simulink model "PubIfDecisionLM_MDL"  (R2020b)
settings: configuration reference "DspaceConfig" (kept outside this file)
PostLoadFcn:
  | if any(exist('dsrtsu_mdlpostloadfcn', 'file') ~= 0), dsrtsu_mdlpostloadfcn('Execute', bdroot); end
InitFcn:
  | , if any(exist('dsmpb_private', 'file') ~= 0), dsmpb_private('dsmpb_mdlclblib', 'Init', bdroot); end,
undefined symbols (not defined in the file or in its folder): OFM_OBJ_FUSIONTYPE_E, OFM_OBJ_MOVINGSTATE_E, OFM_OBJ_ORIENTATION_E, OFM_OBJ_TYPE_E, P_LM_Cyc, P_LM_EMLHistKapRcdBufSize, P_LM_EMLHistTrajBaseDis, P_LM_EMLHistTrajPNum, P_LM_EMLKapCorrMaxThre, P_LM_EMLMinKapThre, P_LM_EMLPathDisDiffThre, P_LM_EMLQuaFiltPar, P_LM_EMLTurnActKapThre, P_LM_EMLValidQuaThre, P_LM_FntPath1Disgap, P_LM_FntPath1MinDis, P_LM_FntPath1Timegap, P_LM_FntPath2Disgap, P_LM_FntPath2MinDis, P_LM_FntPath2Timegap, P_LM_FntPath3Disgap, P_LM_FntPath3MinDis, P_LM_FntPath3Timegap, P_LM_FusBLParFiltP, P_LM_FusEVDifC2Thre, P_LM_FusEVOPath1AllVSLDisThre, P_LM_FusEVOPath1AllVSLLostNumThre, P_LM_FusEVOPath1AllVSLQuaThre, P_LM_FusEVOPath1OTLFacNLC, P_LM_FusOTLQuaThre, P_LM_FusOTLSW, P_LM_FusParC0Index, P_LM_FusParC1Index, P_LM_FusParC2Index, P_LM_FusParC3Index, P_LM_FusVSLQuaThre, P_LM_FusVSLSW, P_LM_FusVSLValidSteerWheerAngThre, P_LM_FusVSLValidVxvThre, P_LM_LaneWidth, P_LM_OTLBufTPInfoEvaFactor, P_LM_OTLObjNum, P_LM_OTLObjSelectAgeThre, P_LM_OTLObjSelectDxAssessVx, P_LM_OTLObjSelectDxThre, P_LM_OTLObjSelectVxThre, P_LM_OTLObjSelectVyAssessDx, P_LM_OTLObjSelectVyThre, P_LM_OTLTrajPntBaseDis, P_LM_OTLTrajStdThre, P_LM_VSLAvailLineNum, P_LM_VSLBLSDiffThre, P_LM_VSLBLSDisRatio, P_LM_VSLFusBLParFiltP_C1, P_LM_VSLFusBLParFiltP_C2, P_LM_VSLFusBLParFiltP_C3, P_LM_VSLFusBLParFiltP_Quality, P_LM_VSLHistTrajBaseDis, P_LM_VSLHistTrajPNum, P_LM_VSLLCC0diff ... (+18)
libraries: simulink x145, LM_LIB x43
(part 19 of 24)

== system PubIfDecisionLM_MDL/Subsystem2/LM_Fusion1/LM_FusRatioCalc/LM_Fusion_EVO/LM_FusEVORatioCalc/LM_Fusion_FntPathK/LM_FusEVOFntPath3/If Action Subsystem1/Subsystem ==
  LM_FusEVOFntPath3EMLFac : Inport
  LM_FusEVOFntPath3VSLFac : Inport  Port=2
  LM_FusEVOFntPath3OTLFac : Inport  Port=3
  LM_EMLFntPath3Quality : Inport  Port=4
  LM_VSLFntPath3Quality : Inport  Port=5
  LM_OTLFntPath3Qulity : Inport  Port=6
  Add : Sum
  Add1 : Sum
  Compare To Zero : simulink/Logic and Bit Operations/Compare To Zero  relop===  OutDataTypeStr=boolean
  Constant : Constant  Value=0.000001  OutDataTypeStr=single
  Divide : Product  Inputs=*/
  Divide1 : Product  Inputs=*/
  Divide2 : Product  Inputs=*/
  Product : Product
  Product1 : Product
  Product2 : Product
  Switch : Switch  Criteria=u2 ~= 0
  LM_FusEVOFntPath3EMLK : Outport
  LM_FusEVOFntPath3VSLK : Outport  Port=2
  LM_FusEVOFntPath3OTLK : Outport  Port=3
  wires:
  Divide1/1 -> LM_FusEVOFntPath3VSLK/1  "LM_FusEVOFntPath3VSLK"
  Divide2/1 -> LM_FusEVOFntPath3OTLK/1  "LM_FusEVOFntPath3OTLK"
  Product/1 -> Divide/1, Add/1
  Add/1 -> Add1/1
  Switch/1 -> Divide2/2, Divide1/2, Divide/2
  Product2/1 -> Divide2/1, Add1/2
  Divide/1 -> LM_FusEVOFntPath3EMLK/1  "LM_FusEVOFntPath3EMLK"
  Product1/1 -> Add/2, Divide1/1
  LM_FusEVOFntPath3OTLFac/1 -> Product2/2
  LM_FusEVOFntPath3VSLFac/1 -> Product1/2
  LM_FusEVOFntPath3EMLFac/1 -> Product/2
  LM_OTLFntPath3Qulity/1 -> Product2/1
  LM_VSLFntPath3Quality/1 -> Product1/1
  LM_EMLFntPath3Quality/1 -> Product/1
  Add1/1 -> Switch/3, Compare To Zero/1
  Compare To Zero/1 -> Switch/2
  Constant/1 -> Switch/1

== system PubIfDecisionLM_MDL/Subsystem2/LM_OTL/LM_OTL_MovObjTrajRecord3/LM_OTL_BufTPCC/Subsystem/LM_OTLHostBufCoordinateConvert/If Action Subsystem/For Each Subsystem/LM_VSL_BufE1Convert ==
  LM_OTLBufE1DxVectK1 : Inport
  LM_OTLBufE1DyVectK1 : Inport  Port=2
  LM_EgoVehOffsetX : Inport  Port=3
  LM_EgoVehOffsetY : Inport  Port=4
  LM_EgoVehOffsetAng : Inport  Port=5
  Add : Sum
  Product{,1..3} (4 alike) : Product
  Sin : Trigonometry
  Sin1 : Trigonometry  Operator=cos
  Subtract : Sum  Inputs=+-
  Subtract1 : Sum  Inputs=+-
  Subtract2 : Sum  Inputs=+-
  LM_OTLBufE1DxVectK1Adju : Outport
  LM_OTLBufE1DyVectK1Adju : Outport  Port=2
  wires:
  Subtract1/1 -> Product3/1, Product1/1
  Sin1/1 -> Product3/2, Product/2
  Product2/1 -> Add/1
  Product/1 -> Subtract2/1
  Product1/1 -> Subtract2/2
  LM_OTLBufE1DyVectK1/1 -> Subtract1/1
  LM_EgoVehOffsetAng/1 -> Sin1/1, Sin/1
  Sin/1 -> Product2/2, Product1/2
  Subtract/1 -> Product2/1, Product/1
  Product3/1 -> Add/2
  Add/1 -> LM_OTLBufE1DyVectK1Adju/1  "LM_OTLBufE1DyVectK1Adju"
  LM_OTLBufE1DxVectK1/1 -> Subtract/1
  LM_EgoVehOffsetY/1 -> Subtract1/2
  LM_EgoVehOffsetX/1 -> Subtract/2
  Subtract2/1 -> LM_OTLBufE1DxVectK1Adju/1  "LM_OTLBufE1DxVectK1Adju"

== system PubIfDecisionLM_MDL/Subsystem2/LM_OTL/LM_OTL_MovObjTrajRecord3/LM_OTL_BufTPCC/Subsystem/LM_OTLHostBufCoordinateConvert/If Action Subsystem/For Each Subsystem/LM_VSL_BufE2Convert ==
  LM_OTLBufE2DxVectK1 : Inport
  LM_OTLBufE2DyVectK1 : Inport  Port=2
  LM_EgoVehOffsetX : Inport  Port=3
  LM_EgoVehOffsetY : Inport  Port=4
  LM_EgoVehOffsetAng : Inport  Port=5
  Add : Sum
  Product{,1..3} (4 alike) : Product
  Sin : Trigonometry
  Sin1 : Trigonometry  Operator=cos
  Subtract : Sum  Inputs=+-
  Subtract1 : Sum  Inputs=+-
  Subtract2 : Sum  Inputs=+-
  LM_OTLBufE2DxVectK1Adju : Outport
  LM_OTLBufE2DyVectK1Adju : Outport  Port=2
  wires:
  Subtract2/1 -> LM_OTLBufE2DxVectK1Adju/1  "LM_OTLBufE2DxVectK1Adju"
  LM_EgoVehOffsetX/1 -> Subtract/2
  LM_EgoVehOffsetY/1 -> Subtract1/2
  LM_OTLBufE2DxVectK1/1 -> Subtract/1
  Add/1 -> LM_OTLBufE2DyVectK1Adju/1  "LM_OTLBufE2DyVectK1Adju"
  Product3/1 -> Add/2
  Subtract/1 -> Product/1, Product2/1
  Sin/1 -> Product1/2, Product2/2
  LM_EgoVehOffsetAng/1 -> Sin/1, Sin1/1
  LM_OTLBufE2DyVectK1/1 -> Subtract1/1
  Product1/1 -> Subtract2/2
  Product/1 -> Subtract2/1
  Product2/1 -> Add/1
  Sin1/1 -> Product/2, Product3/2
  Subtract1/1 -> Product1/1, Product3/1

== system PubIfDecisionLM_MDL/Subsystem2/LM_OTL/LM_OTL_MovObjTrajRecord3/LM_OTL_BufTPCC/Subsystem/LM_OTLLeBufCoordinateConvert/If Action Subsystem/For Each Subsystem/LM_OTL_BufL1Convert ==
  LM_OTLBufL1DxVectK1 : Inport
  LM_OTLBufL1DyVectK1 : Inport  Port=2
  LM_EgoVehOffsetX : Inport  Port=3
  LM_EgoVehOffsetY : Inport  Port=4
  LM_EgoVehOffsetAng : Inport  Port=5
  Add : Sum
  Product{,1..3} (4 alike) : Product
  Sin : Trigonometry
  Sin1 : Trigonometry  Operator=cos
  Subtract : Sum  Inputs=+-
  Subtract1 : Sum  Inputs=+-
  Subtract2 : Sum  Inputs=+-
  LM_OTLBufL1DxVectK1Adju : Outport
  LM_OTLBufL1DyVectK1Adju : Outport  Port=2
  wires:
  Subtract1/1 -> Product3/1, Product1/1
  Sin1/1 -> Product3/2, Product/2
  Product2/1 -> Add/1
  Product/1 -> Subtract2/1
  Product1/1 -> Subtract2/2
  LM_OTLBufL1DyVectK1/1 -> Subtract1/1
  LM_EgoVehOffsetAng/1 -> Sin1/1, Sin/1
  Sin/1 -> Product2/2, Product1/2
  Subtract/1 -> Product2/1, Product/1
  Product3/1 -> Add/2
  Add/1 -> LM_OTLBufL1DyVectK1Adju/1  "LM_OTLBufL1DyVectK1Adju"
  LM_OTLBufL1DxVectK1/1 -> Subtract/1
  LM_EgoVehOffsetY/1 -> Subtract1/2
  LM_EgoVehOffsetX/1 -> Subtract/2
  Subtract2/1 -> LM_OTLBufL1DxVectK1Adju/1  "LM_OTLBufL1DxVectK1Adju"

== system PubIfDecisionLM_MDL/Subsystem2/LM_OTL/LM_OTL_MovObjTrajRecord3/LM_OTL_BufTPCC/Subsystem/LM_OTLLeBufCoordinateConvert/If Action Subsystem/For Each Subsystem/LM_VSL_BufL2Convert ==
  LM_OTLBufL2DxVectK1 : Inport
  LM_OTLBufL2DyVectK1 : Inport  Port=2
  LM_EgoVehOffsetX : Inport  Port=3
  LM_EgoVehOffsetY : Inport  Port=4
  LM_EgoVehOffsetAng : Inport  Port=5
  Add : Sum
  Product{,1..3} (4 alike) : Product
  Sin : Trigonometry
  Sin1 : Trigonometry  Operator=cos
  Subtract : Sum  Inputs=+-
  Subtract1 : Sum  Inputs=+-
  Subtract2 : Sum  Inputs=+-
  LM_OTLBufL2DxVectK1Adju : Outport
  LM_OTLBufL2DyVectK1Adju : Outport  Port=2
  wires:
  Subtract2/1 -> LM_OTLBufL2DxVectK1Adju/1  "LM_OTLBufL2DxVectK1Adju"
  LM_EgoVehOffsetX/1 -> Subtract/2
  LM_EgoVehOffsetY/1 -> Subtract1/2
  LM_OTLBufL2DxVectK1/1 -> Subtract/1
  Add/1 -> LM_OTLBufL2DyVectK1Adju/1  "LM_OTLBufL2DyVectK1Adju"
  Product3/1 -> Add/2
  Subtract/1 -> Product/1, Product2/1
  Sin/1 -> Product1/2, Product2/2
  LM_EgoVehOffsetAng/1 -> Sin/1, Sin1/1
  LM_OTLBufL2DyVectK1/1 -> Subtract1/1
  Product1/1 -> Subtract2/2
  Product/1 -> Subtract2/1
  Product2/1 -> Add/1
  Sin1/1 -> Product/2, Product3/2
  Subtract1/1 -> Product1/1, Product3/1

== system PubIfDecisionLM_MDL/Subsystem2/LM_OTL/LM_OTL_MovObjTrajRecord3/LM_OTL_BufTPCC/Subsystem/LM_OTLRiBufCoordinateConvert/If Action Subsystem/For Each Subsystem/LM_VSL_BufR1Convert ==
  LM_OTLBufR1DxVectK1 : Inport
  LM_OTLBufR1DyVectK1 : Inport  Port=2
  LM_EgoVehOffsetX : Inport  Port=3
  LM_EgoVehOffsetY : Inport  Port=4
  LM_EgoVehOffsetAng : Inport  Port=5
  Add : Sum
  Product{,1..3} (4 alike) : Product
  Sin : Trigonometry
  Sin1 : Trigonometry  Operator=cos
  Subtract : Sum  Inputs=+-
  Subtract1 : Sum  Inputs=+-
  Subtract2 : Sum  Inputs=+-
  LM_OTLBufR1DxVectK1Adju : Outport
  LM_OTLBufR1DyVectK1Adju : Outport  Port=2
  wires:
  Subtract1/1 -> Product3/1, Product1/1
  Sin1/1 -> Product3/2, Product/2
  Product2/1 -> Add/1
  Product/1 -> Subtract2/1
  Product1/1 -> Subtract2/2
  LM_OTLBufR1DyVectK1/1 -> Subtract1/1
  LM_EgoVehOffsetAng/1 -> Sin1/1, Sin/1
  Sin/1 -> Product2/2, Product1/2
  Subtract/1 -> Product2/1, Product/1
  Product3/1 -> Add/2
  Add/1 -> LM_OTLBufR1DyVectK1Adju/1  "LM_OTLBufR1DyVectK1Adju"
  LM_OTLBufR1DxVectK1/1 -> Subtract/1
  LM_EgoVehOffsetY/1 -> Subtract1/2
  LM_EgoVehOffsetX/1 -> Subtract/2
  Subtract2/1 -> LM_OTLBufR1DxVectK1Adju/1  "LM_OTLBufR1DxVectK1Adju"

== system PubIfDecisionLM_MDL/Subsystem2/LM_OTL/LM_OTL_MovObjTrajRecord3/LM_OTL_BufTPCC/Subsystem/LM_OTLRiBufCoordinateConvert/If Action Subsystem/For Each Subsystem/LM_VSL_BufR2Convert ==
  LM_OTLBufR2DxVectK1 : Inport
  LM_OTLBufR2DyVectK1 : Inport  Port=2
  LM_EgoVehOffsetX : Inport  Port=3
  LM_EgoVehOffsetY : Inport  Port=4
  LM_EgoVehOffsetAng : Inport  Port=5
  Add : Sum
  Product{,1..3} (4 alike) : Product
  Sin : Trigonometry
  Sin1 : Trigonometry  Operator=cos
  Subtract : Sum  Inputs=+-
  Subtract1 : Sum  Inputs=+-
  Subtract2 : Sum  Inputs=+-
  LM_OTLBufR2DxVectK1Adju : Outport
  LM_OTLBufR2DyVectK1Adju : Outport  Port=2
  wires:
  Subtract2/1 -> LM_OTLBufR2DxVectK1Adju/1  "LM_OTLBufR2DxVectK1Adju"
  LM_EgoVehOffsetX/1 -> Subtract/2
  LM_EgoVehOffsetY/1 -> Subtract1/2
  LM_OTLBufR2DxVectK1/1 -> Subtract/1
  Add/1 -> LM_OTLBufR2DyVectK1Adju/1  "LM_OTLBufR2DyVectK1Adju"
  Product3/1 -> Add/2
  Subtract/1 -> Product/1, Product2/1
  Sin/1 -> Product1/2, Product2/2
  LM_EgoVehOffsetAng/1 -> Sin/1, Sin1/1
  LM_OTLBufR2DyVectK1/1 -> Subtract1/1
  Product1/1 -> Subtract2/2
  Product/1 -> Subtract2/1
  Product2/1 -> Add/1
  Sin1/1 -> Product/2, Product3/2
  Subtract1/1 -> Product1/1, Product3/1

== system PubIfDecisionLM_MDL/Subsystem2/LM_OTL/LM_OTL_MovObjTrajRecord3/LM_OTL_MovObjSelc/LM_OTL_MovObjInterestedSelc/LM_OTL_ObjSelcIndexCalc/LM_OTL_ObjSelcCalc/LM_OTL_HostObjSelc/LM_OTL_HostObj1Selc ==
  C_LM_ObjNum : Inport
  In4 : Inport  Port=2
  Compare To Constant : simulink/Logic and Bit Operations/Compare To Constant  relop===  const=1  OutDataTypeStr=boolean
  Relational Operator : RelationalOperator  Operator=<  OutDataTypeStr=boolean  RndMeth=Simplest
  Switch : Switch  Criteria=u2 > Threshold
  Switch2 : Switch  Criteria=u2 ~= 0
  Switch28 : Switch  Criteria=u2 ~= 0
  Switch5 : Switch  Criteria=u2 > Threshold
  Unit Delay : UnitDelay  SampleTime=-1  HasFrameUpgradeWarning=on
  Unit Delay2 : UnitDelay  InitialCondition=255  SampleTime=-1  HasFrameUpgradeWarning=on
  LM_OTLHostObj1Index : Outport
  HostObj2SelcTrig : Outport  Port=2
  HostObj2SelcIndexPro : Outport  Port=3
  HostObj2SelcDxPro : Outport  Port=4
  wires:
  Compare To Constant/1 -> Switch28/2, Switch/2
  Relational Operator/1 -> Switch5/2, Switch2/2, HostObj2SelcTrig/1
  Switch28/1 -> Switch2/3
  In4/1 -> Relational Operator/1, Switch5/1, Switch/1
  C_LM_ObjNum/1 -> Compare To Constant/1, Switch2/1, Switch28/1
  Switch/1 -> Unit Delay2/1
  Switch2/1 -> Unit Delay/1, LM_OTLHostObj1Index/1
  Switch5/1 -> Switch/3
  Unit Delay/1 -> HostObj2SelcIndexPro/1, Switch28/3
  Unit Delay2/1 -> Switch5/3, HostObj2SelcDxPro/1, Relational Operator/2

== system PubIfDecisionLM_MDL/Subsystem2/LM_OTL/LM_OTL_MovObjTrajRecord3/LM_OTL_MovObjSelc/LM_OTL_MovObjInterestedSelc/LM_OTL_ObjSelcIndexCalc/LM_OTL_ObjSelcCalc/LM_OTL_HostObjSelc/LM_OTL_HostObj2Selc ==
  HostObj2SelcTrig : Inport
  HostObj2SelcIndexPro : Inport  Port=2
  HostObj2SelcDxPro : Inport  Port=3
  LM_OTL_HostObjSelcDxInfo : Inport  Port=4
  C_LM_ObjNum : Inport  Port=5
  Compare To Constant : simulink/Logic and Bit Operations/Compare To Constant  relop===  const=1  OutDataTypeStr=boolean
  Constant10 : Constant  Value=0  OutDataTypeStr=int32
  Constant8 : Constant  Value=255  OutDataTypeStr=single
  Relational Operator3 : RelationalOperator  Operator=<  OutDataTypeStr=boolean  RndMeth=Simplest
  Switch{20..22,26..27} (5 alike) : Switch  Criteria=u2 > Threshold
  Switch3 : Switch  Criteria=u2 ~= 0
  Unit Delay1 : UnitDelay  SampleTime=-1  HasFrameUpgradeWarning=on
  Unit Delay9 : UnitDelay  InitialCondition=255  SampleTime=-1  HasFrameUpgradeWarning=on
  LM_OTLLeObj2Index : Outport
  wires:
  HostObj2SelcDxPro/1 -> Switch20/1
  HostObj2SelcIndexPro/1 -> Switch3/1
  Constant10/1 -> Switch26/1
  Switch20/1 -> Switch21/3
  Switch27/1 -> Switch3/3
  Unit Delay1/1 -> Switch27/3
  Switch3/1 -> Switch26/3
  Unit Delay9/1 -> Switch22/3, Relational Operator3/2
  Constant8/1 -> Switch21/1
  HostObj2SelcTrig/1 -> Switch3/2, Switch20/2
  Relational Operator3/1 -> Switch22/2, Switch27/2
  C_LM_ObjNum/1 -> Switch27/1, Compare To Constant/1
  Switch26/1 -> LM_OTLLeObj2Index/1, Unit Delay1/1
  Compare To Constant/1 -> Switch26/2, Switch21/2
  Switch21/1 -> Unit Delay9/1
  LM_OTL_HostObjSelcDxInfo/1 -> Relational Operator3/1, Switch22/1
  Switch22/1 -> Switch20/3

== system PubIfDecisionLM_MDL/Subsystem2/LM_OTL/LM_OTL_MovObjTrajRecord3/LM_OTL_MovObjSelc/LM_OTL_MovObjInterestedSelc/LM_OTL_ObjSelcIndexCalc/LM_OTL_ObjSelcCalc/LM_OTL_LeObjSelc/LM_OTL_LeObj1Selc ==
  C_LM_ObjNum : Inport
  LeObjSelcDxInfo : Inport  Port=2
  Compare To Constant : simulink/Logic and Bit Operations/Compare To Constant  relop===  const=1  OutDataTypeStr=boolean
  Relational Operator : RelationalOperator  Operator=<  OutDataTypeStr=boolean  RndMeth=Simplest
  Switch : Switch  Criteria=u2 > Threshold
  Switch2 : Switch  Criteria=u2 ~= 0
  Switch28 : Switch  Criteria=u2 ~= 0
  Switch5 : Switch  Criteria=u2 > Threshold
  Unit Delay : UnitDelay  SampleTime=-1  HasFrameUpgradeWarning=on
  Unit Delay2 : UnitDelay  InitialCondition=255  SampleTime=-1  HasFrameUpgradeWarning=on
  LM_OTLLeObj1Index : Outport
  LeObj2SelcTrig : Outport  Port=2
  LeObj2SelcIndexPro : Outport  Port=3
  LeObj2SelcDxPro : Outport  Port=4
  wires:
  Compare To Constant/1 -> Switch28/2, Switch/2
  Relational Operator/1 -> Switch5/2, Switch2/2, LeObj2SelcTrig/1
  Switch28/1 -> Switch2/3
  LeObjSelcDxInfo/1 -> Relational Operator/1, Switch5/1, Switch/1
  C_LM_ObjNum/1 -> Switch2/1, Switch28/1, Compare To Constant/1
  Switch/1 -> Unit Delay2/1
  Switch2/1 -> Unit Delay/1, LM_OTLLeObj1Index/1
  Switch5/1 -> Switch/3
  Unit Delay/1 -> LeObj2SelcIndexPro/1, Switch28/3
  Unit Delay2/1 -> Switch5/3, LeObj2SelcDxPro/1, Relational Operator/2

== system PubIfDecisionLM_MDL/Subsystem2/LM_OTL/LM_OTL_MovObjTrajRecord3/LM_OTL_MovObjSelc/LM_OTL_MovObjInterestedSelc/LM_OTL_ObjSelcIndexCalc/LM_OTL_ObjSelcCalc/LM_OTL_LeObjSelc/LM_OTL_LeObj2Selc ==
  LeObj2SelcTrig : Inport
  LeObj2SelcIndexPro : Inport  Port=2
  LeObj2SelcDxPro : Inport  Port=3
  LeObjSelcDxInfo : Inport  Port=4
  C_LM_ObjNum : Inport  Port=5
  Compare To Constant : simulink/Logic and Bit Operations/Compare To Constant  relop===  const=1  OutDataTypeStr=boolean
  Constant10 : Constant  Value=0  OutDataTypeStr=int32
  Constant8 : Constant  Value=255  OutDataTypeStr=single
  Relational Operator3 : RelationalOperator  Operator=<  OutDataTypeStr=boolean  RndMeth=Simplest
  Switch{20..22,26..27} (5 alike) : Switch  Criteria=u2 > Threshold
  Switch3 : Switch  Criteria=u2 ~= 0
  Unit Delay1 : UnitDelay  SampleTime=-1  HasFrameUpgradeWarning=on
  Unit Delay9 : UnitDelay  InitialCondition=255  SampleTime=-1  HasFrameUpgradeWarning=on
  LM_OTLLeObj2Index : Outport
  wires:
  LeObj2SelcDxPro/1 -> Switch20/1
  LeObj2SelcIndexPro/1 -> Switch3/1
  Constant10/1 -> Switch26/1
  Switch20/1 -> Switch21/3
  Switch27/1 -> Switch3/3
  Unit Delay1/1 -> Switch27/3
  Switch3/1 -> Switch26/3
  Unit Delay9/1 -> Switch22/3, Relational Operator3/2
  Constant8/1 -> Switch21/1
  LeObj2SelcTrig/1 -> Switch20/2, Switch3/2
  Relational Operator3/1 -> Switch22/2, Switch27/2
  C_LM_ObjNum/1 -> Switch27/1, Compare To Constant/1
  Switch26/1 -> LM_OTLLeObj2Index/1, Unit Delay1/1
  Compare To Constant/1 -> Switch26/2, Switch21/2
  Switch21/1 -> Unit Delay9/1
  LeObjSelcDxInfo/1 -> Relational Operator3/1, Switch22/1
  Switch22/1 -> Switch20/3

== system PubIfDecisionLM_MDL/Subsystem2/LM_OTL/LM_OTL_MovObjTrajRecord3/LM_OTL_MovObjSelc/LM_OTL_MovObjInterestedSelc/LM_OTL_ObjSelcIndexCalc/LM_OTL_ObjSelcCalc/LM_OTL_RigObjSelc/LM_OTL_RigObj1Selc ==
  C_LM_ObjNum : Inport
  In4 : Inport  Port=2
  Compare To Constant : simulink/Logic and Bit Operations/Compare To Constant  relop===  const=1  OutDataTypeStr=boolean
  Relational Operator : RelationalOperator  Operator=<  OutDataTypeStr=boolean  RndMeth=Simplest
  Switch : Switch  Criteria=u2 > Threshold
  Switch2 : Switch  Criteria=u2 ~= 0
  Switch28 : Switch  Criteria=u2 ~= 0
  Switch5 : Switch  Criteria=u2 > Threshold
  Unit Delay : UnitDelay  SampleTime=-1  HasFrameUpgradeWarning=on
  Unit Delay2 : UnitDelay  InitialCondition=255  SampleTime=-1  HasFrameUpgradeWarning=on
  LM_OTLLeObj1Index : Outport
  RigObj2SelcTrig : Outport  Port=2
  RigObj2SelcIndexPro : Outport  Port=3
  RigObj2SelcDxPro : Outport  Port=4
  wires:
  Compare To Constant/1 -> Switch28/2, Switch/2
  Relational Operator/1 -> Switch5/2, RigObj2SelcTrig/1, Switch2/2
  Switch28/1 -> Switch2/3
  In4/1 -> Switch5/1, Switch/1, Relational Operator/1
  C_LM_ObjNum/1 -> Compare To Constant/1, Switch2/1, Switch28/1
  Switch/1 -> Unit Delay2/1
  Switch2/1 -> Unit Delay/1, LM_OTLLeObj1Index/1
  Switch5/1 -> Switch/3
  Unit Delay/1 -> RigObj2SelcIndexPro/1, Switch28/3
  Unit Delay2/1 -> Switch5/3, RigObj2SelcDxPro/1, Relational Operator/2

== system PubIfDecisionLM_MDL/Subsystem2/LM_OTL/LM_OTL_MovObjTrajRecord3/LM_OTL_MovObjSelc/LM_OTL_MovObjInterestedSelc/LM_OTL_ObjSelcIndexCalc/LM_OTL_ObjSelcCalc/LM_OTL_RigObjSelc/LM_OTL_RigObj2Selc ==
  RigObj2SelcTrig : Inport
  RigObj2SelcIndexPro : Inport  Port=2
  RigObj2SelcDxPro : Inport  Port=3
  LM_OTL_RigObjSelcDxInfo : Inport  Port=4
  C_LM_ObjNum : Inport  Port=5
  Compare To Constant : simulink/Logic and Bit Operations/Compare To Constant  relop===  const=1  OutDataTypeStr=boolean
  Constant10 : Constant  Value=0  OutDataTypeStr=int32
  Constant8 : Constant  Value=255  OutDataTypeStr=single
  Relational Operator3 : RelationalOperator  Operator=<  OutDataTypeStr=boolean  RndMeth=Simplest
  Switch{20..22,26..27} (5 alike) : Switch  Criteria=u2 > Threshold
  Switch3 : Switch  Criteria=u2 ~= 0
  Unit Delay1 : UnitDelay  SampleTime=-1  HasFrameUpgradeWarning=on
  Unit Delay9 : UnitDelay  InitialCondition=255  SampleTime=-1  HasFrameUpgradeWarning=on
  LM_OTLLeObj2Index : Outport
  wires:
  RigObj2SelcDxPro/1 -> Switch20/1
  RigObj2SelcIndexPro/1 -> Switch3/1
  Constant10/1 -> Switch26/1
  Switch20/1 -> Switch21/3
  Switch27/1 -> Switch3/3
  Unit Delay1/1 -> Switch27/3
  Switch3/1 -> Switch26/3
  Unit Delay9/1 -> Switch22/3, Relational Operator3/2
  Constant8/1 -> Switch21/1
  RigObj2SelcTrig/1 -> Switch3/2, Switch20/2
  Relational Operator3/1 -> Switch22/2, Switch27/2
  C_LM_ObjNum/1 -> Switch27/1, Compare To Constant/1
  Switch26/1 -> LM_OTLLeObj2Index/1, Unit Delay1/1
  Compare To Constant/1 -> Switch26/2, Switch21/2
  Switch21/1 -> Unit Delay9/1
  LM_OTL_RigObjSelcDxInfo/1 -> Relational Operator3/1, Switch22/1
  Switch22/1 -> Switch20/3

== system PubIfDecisionLM_MDL/Subsystem2/LM_VSL/LM_VSLFntPath/LM_VSL_LineInfoEvalutaion/LM_VSL_BaseLinePCalc3/Subsystem/Switch Case Action Subsystem/LM_VSLLineQualitySumCalc/Subsystem ==
  LM_VSLLineDisFntVect : Inport
  LM_VSLBLFntDis : Inport  Port=2
  If : If  IfExpression=u1 > 40
  If Action Subsystem : Subsystem  TreatAsAtomicUnit=on
  If Action Subsystem1 : Subsystem  TreatAsAtomicUnit=on
  Merge : Merge
  LM_VSLFntDisValid : Outport
  wires:
  Merge/1 -> LM_VSLFntDisValid/1
  If/1 -> If Action Subsystem1/Action
  LM_VSLLineDisFntVect/1 -> If Action Subsystem/1(LM_VSLLineDisFnt), If/1
  If Action Subsystem/1(LM_VSLFntDisValid) -> Merge/2
  If/2 -> If Action Subsystem/Action
  LM_VSLBLFntDis/1 -> If Action Subsystem/2(LM_VSLBLFntDis)
  If Action Subsystem1/1(LM_VSLFntDisValid) -> Merge/1

== system PubIfDecisionLM_MDL/Subsystem2/LM_VSL/LM_VSLFntPath/LM_VSL_LineInfoEvalutaion/LM_VSL_BaseLinePCalc3/Subsystem/Switch Case Action Subsystem/LM_VSLLineQualitySumCalc/Subsystem/If Action Subsystem ==
  LM_VSLLineDisFnt : Inport
  LM_VSLBLFntDis : Inport  Port=2
  Action Port : ActionPort  ActionPortLabel=else
  Constant : Constant  Value=P_LM_VSLBLSDisRatio
  Product : Product
  Relational Operator : RelationalOperator  OutDataTypeStr=boolean  RndMeth=Simplest
  LM_VSLFntDisValid : Outport
  wires:
  Constant/1 -> Product/2
  Relational Operator/1 -> LM_VSLFntDisValid/1
  Product/1 -> Relational Operator/2
  LM_VSLBLFntDis/1 -> Product/1
  LM_VSLLineDisFnt/1 -> Relational Operator/1

== system PubIfDecisionLM_MDL/Subsystem2/LM_VSL/LM_VSLFntPath/LM_VSL_LineInfoEvalutaion/LM_VSL_BaseLinePCalc3/Subsystem/Switch Case Action Subsystem/LM_VSLLineQualitySumCalc/Subsystem/If Action Subsystem1 ==
  Action Port : ActionPort  ActionPortLabel=if(u1 > 40)
  Constant : Constant  Value=true  OutDataTypeStr=boolean
  LM_VSLFntDisValid : Outport
  wires:
  Constant/1 -> LM_VSLFntDisValid/1

== matlab function PubIfDecisionLM_MDL/Subsystem2/LM_VSL/LM_VSLRearPath/LM_VSLHistLineInfoRcdBufferUpdate/MATLAB Function1 ==
  data: LM_VSLLRC0HistInfox input; LM_VSLLRC0HistInfoX output; LM_VSLLRC0HistInfoy input; LM_VSLRLC0HistInfox input; LM_VSLRLC0HistInfoy input; LM_VSLHistLineInfoRcdFlg input; LM_EMLHistPEndPos input; LM_VSLLaChgC0JumpFlg input; LM_VSLLRC0HistInfoY output; LM_VSLRLC0HistInfoX output; LM_VSLRLC0HistInfoY output
function [LM_VSLLRC0HistInfoX,LM_VSLLRC0HistInfoY,LM_VSLRLC0HistInfoX,LM_VSLRLC0HistInfoY] = fcn(LM_VSLLRC0HistInfox,LM_VSLLRC0HistInfoy,LM_VSLRLC0HistInfox,LM_VSLRLC0HistInfoy,LM_VSLHistLineInfoRcdFlg, LM_EMLHistPEndPos,LM_VSLLaChgC0JumpFlg)
%%
%%
% LM_VSLLRC0HistInfoX = LM_VSLLRC0HistInfox;
% LM_VSLLRC0HistInfoY = LM_VSLLRC0HistInfoy;
% LM_VSLRLC0HistInfoX = LM_VSLRLC0HistInfox;
% LM_VSLRLC0HistInfoY = LM_VSLRLC0HistInfoy;
% tag = LM_EMLHistPEndPos - uint8(1);
% if LM_EMLHistPEndPos == uint8(1)
%     tag = uint8(60);
% end
%  if sign == 1
%      x_deviation = LM_VSLLRC0HistInfox(tag) - LM_VSLRLC0HistInfox(tag);
%      y_deviation = LM_VSLLRC0HistInfoy(tag) - LM_VSLRLC0HistInfoy(tag);
%      t1 = LM_VSLLRC0HistInfoy(LM_EMLHistPEndPos);
%      t2 = LM_VSLLRC0HistInfoy(tag);
%      t3 = t1 - t2;
%      t4 = LM_VSLRLC0HistInfoy(tag);
%      t5 = LM_VSLRLC0HistInfoy(LM_EMLHistPEndPos);
%      t6 = t4 - t5;
%      if LM_VSLLRC0HistInfoy(LM_EMLHistPEndPos)-LM_VSLLRC0HistInfoy(tag)>1.75 
%          LM_VSLRLC0HistInfoX = LM_VSLRLC0HistInfox + x_deviation;
%          LM_VSLRLC0HistInfoY = LM_VSLRLC0HistInfoy + y_deviation;
%          LM_VSLRLC0HistInfoX(LM_EMLHistPEndPos) = LM_VSLRLC0HistInfox(LM_EMLHistPEndPos);
%          LM_VSLRLC0HistInfoY(LM_EMLHistPEndPos) = LM_VSLRLC0HistInfoy(LM_EMLHistPEndPos);
%          LM_VSLLRC0HistInfoX = LM_VSLLRC0HistInfox;
%          LM_VSLLRC0HistInfoY = 3.5 - LM_VSLRLC0HistInfoY;
%      elseif LM_VSLRLC0HistInfoy(tag)-LM_VSLRLC0HistInfoy(LM_EMLHistPEndPos)>1.75 
%          LM_VSLLRC0HistInfoX = LM_VSLLRC0HistInfox - x_deviation;
%          LM_VSLLRC0HistInfoY = LM_VSLLRC0HistInfoy - y_deviation;
%          LM_VSLLRC0HistInfoX(LM_EMLHistPEndPos) = LM_VSLLRC0HistInfox(LM_EMLHistPEndPos);
%          LM_VSLLRC0HistInfoY(LM_EMLHistPEndPos) = LM_VSLLRC0HistInfoy(LM_EMLHistPEndPos);
%          LM_VSLRLC0HistInfoX = LM_VSLRLC0HistInfox;
%          LM_VSLRLC0HistInfoY = 3.5 - LM_VSLRLC0HistInfoy;
%      else
%          LM_VSLLRC0HistInfoX = LM_VSLLRC0HistInfox;
%          LM_VSLLRC0HistInfoY = LM_VSLLRC0HistInfoy;
%          LM_VSLRLC0HistInfoX = LM_VSLRLC0HistInfox;
%          LM_VSLRLC0HistInfoY = LM_VSLRLC0HistInfoy;
%      end
             
LM_VSLLRC0HistInfoX = LM_VSLLRC0HistInfox;
LM_VSLLRC0HistInfoY = LM_VSLLRC0HistInfoy;
LM_VSLRLC0HistInfoX = LM_VSLRLC0HistInfox;
LM_VSLRLC0HistInfoY = LM_VSLRLC0HistInfoy;
tag = LM_EMLHistPEndPos - uint8(1);
if LM_EMLHistPEndPos == uint8(1)
    tag = uint8(60);
end

 if LM_VSLLaChgC0JumpFlg ~= 0
     if LM_VSLLaChgC0JumpFlg == 1 % 左换道
         % 暂存跳变后c0信息
         t_L1C0EndX = LM_VSLLRC0HistInfox(tag);
         t_L1C0EndY = LM_VSLLRC0HistInfoy(LM_EMLHistPEndPos);
         t_R1C0EndX = LM_VSLRLC0HistInfox(tag);
         t_R1C0EndY = LM_VSLRLC0HistInfoy(LM_EMLHistPEndPos);
         % 计算偏移量
         offset_x = t_L1C0EndX - t_R1C0EndX;
         offset_y = t_L1C0EndY - t_R1C0EndY;
         % 轨迹点偏移
         LM_VSLLRC0HistInfoX = LM_VSLLRC0HistInfox + offset_x;
         LM_VSLLRC0HistInfoY = LM_VSLLRC0HistInfoy + offset_y;
         if LM_VSLHistLineInfoRcdFlg == true
             LM_VSLLRC0HistInfoX(LM_EMLHistPEndPos) = LM_VSLLRC0HistInfox(LM_EMLHistPEndPos);
             LM_VSLLRC0HistInfoY(LM_EMLHistPEndPos) = t_L1C0EndY;
         end
         LM_VSLRLC0HistInfoX = LM_VSLLRC0HistInfox;
         LM_VSLRLC0HistInfoY = LM_VSLLRC0HistInfoy;
         if LM_VSLHistLineInfoRcdFlg == true
             LM_VSLRLC0HistInfoX(LM_EMLHistPEndPos) = LM_VSLRLC0HistInfox(LM_EMLHistPEndPos);
             LM_VSLRLC0HistInfoY(LM_EMLHistPEndPos) = t_R1C0EndY;
         end
     else %右换道 
         % 暂存跳变后c0信息
         t_L1C0EndX = LM_VSLLRC0HistInfox(tag);
         t_L1C0EndY = LM_VSLLRC0HistInfoy(LM_EMLHistPEndPos);
         t_R1C0EndX = LM_VSLRLC0HistInfox(tag);
         t_R1C0EndY = LM_VSLRLC0HistInfoy(LM_EMLHistPEndPos);
         % 计算偏移量
         offset_x = t_R1C0EndX - t_L1C0EndX;
         offset_y = t_R1C0EndY - t_L1C0EndY;
         
         LM_VSLRLC0HistInfoX = LM_VSLRLC0HistInfox + offset_x;
         LM_VSLRLC0HistInfoY = LM_VSLRLC0HistInfoy + offset_y;
         if LM_VSLHistLineInfoRcdFlg == true
             LM_VSLRLC0HistInfoX(LM_EMLHistPEndPos) = LM_VSLRLC0HistInfox(LM_EMLHistPEndPos);
             LM_VSLRLC0HistInfoY(LM_EMLHistPEndPos) = t_R1C0EndY;
         end
         LM_VSLLRC0HistInfoX = LM_VSLRLC0HistInfox;
         LM_VSLLRC0HistInfoY = LM_VSLRLC0HistInfoy;
         if LM_VSLHistLineInfoRcdFlg == true
             LM_VSLLRC0HistInfoX(LM_EMLHistPEndPos) = LM_VSLLRC0HistInfox(LM_EMLHistPEndPos);
             LM_VSLLRC0HistInfoY(LM_EMLHistPEndPos) = t_L1C0EndY;
         end
     end
 end
end

== matlab function PubIfDecisionLM_MDL/Subsystem2/LM_VSL/LM_VSLRearPath/LM_VSLHistLineInfoRcdBufferUpdate/MATLAB Function2 ==
  data: LM_VSLHistPEndPos input; LM_VSLLLC0HistInfoX output; LM_VSLLLC0HistInfoXK1Adju input
function LM_VSLLLC0HistInfoX = fcn(LM_VSLHistPEndPos,LM_VSLLLC0HistInfoXK1Adju)

LM_VSLLLC0HistInfoX = LM_VSLLLC0HistInfoXK1Adju;
LM_VSLLLC0HistInfoX(LM_VSLHistPEndPos) = single(0);

== matlab function PubIfDecisionLM_MDL/Subsystem2/LM_VSL/LM_VSLRearPath/LM_VSLHistLineInfoRcdBufferUpdate/MATLAB Function3 ==
  data: LM_VSLHistPEndPos input; LM_VSLLLC0HistInfoY output; LM_VSLLLC0HistInfoYK1Adju input; LM_VSLLRC0 input; LM_VSLLaChgC0JumpFlg input
function LM_VSLLLC0HistInfoY = fcn(LM_VSLHistPEndPos,LM_VSLLLC0HistInfoYK1Adju,LM_VSLLRC0,LM_VSLLaChgC0JumpFlg)

LM_VSLLLC0HistInfoY = LM_VSLLLC0HistInfoYK1Adju;
if LM_VSLLaChgC0JumpFlg == uint8(0)
    if LM_VSLHistPEndPos ~= 1
        t_c0k1 = LM_VSLLLC0HistInfoY(LM_VSLHistPEndPos-1);
    else 
        t_c0k1 = LM_VSLLLC0HistInfoY(60);
    end
    if abs(LM_VSLLRC0 - t_c0k1) > 1
        t_c0 = t_c0k1 + single(0.25) * (LM_VSLLRC0 - t_c0k1);
    else
        t_c0 = LM_VSLLRC0;
    end
else
    t_c0 = LM_VSLLRC0;
end
% t_c0 = LM_VSLLRC0;
LM_VSLLLC0HistInfoY(LM_VSLHistPEndPos) = single(t_c0);

== matlab function PubIfDecisionLM_MDL/Subsystem2/LM_VSL/LM_VSLRearPath/LM_VSLHistLineInfoRcdBufferUpdate/MATLAB Function4 ==
  data: LM_VSLHistPEndPos input; LM_VSLLLC0HistInfoX output; LM_VSLLLC0HistInfoXK1Adju input
function LM_VSLLLC0HistInfoX = fcn(LM_VSLHistPEndPos,LM_VSLLLC0HistInfoXK1Adju)

LM_VSLLLC0HistInfoX = LM_VSLLLC0HistInfoXK1Adju;
LM_VSLLLC0HistInfoX(LM_VSLHistPEndPos) = single(0);

== matlab function PubIfDecisionLM_MDL/Subsystem2/LM_VSL/LM_VSLRearPath/LM_VSLHistLineInfoRcdBufferUpdate/MATLAB Function5 ==
  data: LM_VSLHistPEndPos input; LM_VSLLLC0HistInfoY output; LM_VSLLLC0HistInfoYK1Adju input; LM_VSLRLC0 input; LM_VSLLaChgC0JumpFlg input
function LM_VSLLLC0HistInfoY = fcn(LM_VSLHistPEndPos,LM_VSLLLC0HistInfoYK1Adju,LM_VSLRLC0,LM_VSLLaChgC0JumpFlg)

LM_VSLLLC0HistInfoY = LM_VSLLLC0HistInfoYK1Adju;
if LM_VSLLaChgC0JumpFlg == uint8(0)
    if LM_VSLHistPEndPos ~= 1
        t_c0k1 = LM_VSLLLC0HistInfoY(LM_VSLHistPEndPos-1);
    else 
        t_c0k1 = LM_VSLLLC0HistInfoY(60);
    end
    if abs(LM_VSLRLC0 - t_c0k1) > 1
        t_c0 = t_c0k1 + single(0.25) * (LM_VSLRLC0 - t_c0k1);
    else
        t_c0 = LM_VSLRLC0;
    end
else
    t_c0 = LM_VSLRLC0;
end
% t_c0 = t_c0k1 + single(0.25) * (LM_VSLRLC0 - t_c0k1);
LM_VSLLLC0HistInfoY(LM_VSLHistPEndPos) = single(t_c0);

== matlab function PubIfDecisionLM_MDL/Subsystem2/LM_VSL/LM_VSLRearPath/MATLAB Function1 ==
  data: LM_VSLLRC0HistInfoX input; LM_VSLRearPath1P output; LM_VSLLRC0HistInfoY input; LM_VSLRLC0HistInfoX input; LM_VSLRLC0HistInfoY input; LM_VSLHistPNum input; LM_EMLHistPEndPos input; LM_EMLHistPFristPos input; LM_RearPath1Dis input; LM_RearPath2Dis input; LM_RearPath3Dis input; LM_VSLRearPath1Qulity output; LM_VSLRearPath2P output; LM_VSLRearPath2Qulity output; LM_VSLRearPath3P output; LM_VSLRearPath3Qulity output; P_LM_VSLRearLaneQualityRatio input; P_LM_VSLRearLanePolyfitQualityRatio input
 function [LM_VSLRearPath1P,LM_VSLRearPath1Qulity,LM_VSLRearPath2P,LM_VSLRearPath2Qulity,LM_VSLRearPath3P,LM_VSLRearPath3Qulity] = ...
    fcn(LM_VSLLRC0HistInfoX,LM_VSLLRC0HistInfoY,LM_VSLRLC0HistInfoX,LM_VSLRLC0HistInfoY,LM_VSLHistPNum,LM_EMLHistPEndPos,LM_EMLHistPFristPos,LM_RearPath1Dis,LM_RearPath2Dis,LM_RearPath3Dis,P_LM_VSLRearLaneQualityRatio,P_LM_VSLRearLanePolyfitQualityRatio)
%初始化拟合用dx,dy buffer 
 P_LM_EMLHistPNum = 60;
t_index = uint8(zeros(1,P_LM_EMLHistPNum));
if LM_VSLHistPNum > P_LM_EMLHistPNum
     if LM_EMLHistPEndPos == 1
        t_index(1) = uint8(1);
        for i = 2:P_LM_EMLHistPNum
            t_index(i) = uint8(P_LM_EMLHistPNum+2-i);
        end
    elseif LM_EMLHistPEndPos == P_LM_EMLHistPNum
        for i = 1:P_LM_EMLHistPNum
            t_index(i) = uint8(P_LM_EMLHistPNum+1-i);
        end
    else
        for i = 1:P_LM_EMLHistPNum
            if i <= LM_EMLHistPEndPos
                t_index(i) = uint8(LM_EMLHistPEndPos+1-i);
            else
                t_index(i) = uint8(P_LM_EMLHistPNum+1-(i-LM_EMLHistPEndPos));
            end
        end
    end
else
    for i = 1:P_LM_EMLHistPNum
            if i <= LM_EMLHistPEndPos
                t_index(i) = uint8(LM_EMLHistPEndPos+1-i);
            else
                t_index(i) = 1;
            end
    end
end

%% 后方一段轨迹拟合
Tag=0;
if Tag==0  
   LM_VSLC0BufferDis=single(255);
end
P_LM_EMLHPFitBuffSize = 60;
t_hpx = single(zeros(P_LM_EMLHPFitBuffSize,1));
t_hpy = single(zeros(P_LM_EMLHPFitBuffSize,1));
t_pnum = uint8(0);
if LM_VSLHistPNum > P_LM_EMLHistPNum
    t_fornum = uint8(P_LM_EMLHistPNum);
else
    t_fornum = uint8(LM_VSLHistPNum);
end

y_left = zeros(60,1);
y_right = zeros(60,1);
LM_VSLC0HistInfoX = single(zeros(60,1));
LM_VSLC0HistInfoY = single(zeros(60,1));
if t_fornum >=2
   for u = 1:t_fornum-1
       y_left(u) = abs(LM_VSLLRC0HistInfoY(t_index(u))-LM_VSLLRC0HistInfoY(t_index(u+1)));
       y_right(u) = abs(LM_VSLRLC0HistInfoY(t_index(u))-LM_VSLRLC0HistInfoY(t_index(u+1)));
   end
   mean_L = sum(y_left)/single(u);
   variance_L = sum((y_left(:,1)- mean_L).^2)/single(u);
   mean_R = sum(y_right)/single(u);
   variance_R = sum((y_right(:,1)- mean_R).^2)/single(u);
   variance = min(variance_L,variance_R);
   if variance < P_LM_VSLRearLaneQualityRatio
       if variance == variance_L
           LM_VSLC0HistInfoX = LM_VSLLRC0HistInfoX;
           LM_VSLC0HistInfoY = LM_VSLLRC0HistInfoY;
       else 
           LM_VSLC0HistInfoX = LM_VSLRLC0HistInfoX;
           LM_VSLC0HistInfoY = LM_VSLRLC0HistInfoY;
       end
   else
           LM_VSLC0HistInfoX = 0.5*LM_VSLLRC0HistInfoX+0.5*LM_VSLRLC0HistInfoX;
           LM_VSLC0HistInfoY = 0.5*LM_VSLLRC0HistInfoY+0.5*LM_VSLRLC0HistInfoY;
   end 
end
for i = 1:t_fornum
    if abs(LM_VSLC0HistInfoX(t_index(i))) <= abs(LM_RearPath3Dis)
        t_pnum = t_pnum + 1;
        if LM_VSLC0BufferDis==255
           t_hpx(t_pnum) = LM_VSLC0HistInfoX(t_index(i));
           t_hpy(t_pnum) = LM_VSLC0HistInfoY(t_index(i));
        end
    end
end
if t_pnum ~=0
      if t_pnum < P_LM_EMLHPFitBuffSize 
        for i = t_pnum+1:P_LM_EMLHPFitBuffSize
            t_hpx(i) = t_hpx(t_pnum);
           t_hpy(i) = t_hpy(t_pnum);
        end
      end
      z = single(zeros(3,1));
      I = single(zeros(3,1));
      t_x=single(zeros(20,1));
      t_y=single(zeros(20,1));
      for i=1:20
          z(1) = t_hpx(3*i-2);
          z(2) = t_hpx(3*i-1);
          z(3) = t_hpx(3*i);
          I(1) = t_hpy(3*i-2);
          I(2) = t_hpy(3*i-1);
          I(3) = t_hpy(3*i);
          t_x(i)= median(z);
          t_y(i)= median(I);
      end
     x =t_y;
     t_y = hampel1(x);
    % 第1段参数拟合
    LM_VSLRearPath3P = polyfit(t_x,t_y,3);
    % 第一段拟合误差计算
    t_fity = polyval(LM_VSLRearPath3P,t_x);
    t_sumerry = single(0);
    for i=1:20
        t_erry = single((t_y(i) - t_fity(i))^2);
        t_sumerry = t_sumerry + t_erry;
    end
    if t_sumerry < P_LM_VSLRearLanePolyfitQualityRatio
    t_quality = interpolate(single(0.5),single(1),single(3),single(0),single(t_sumerry));
    t_factor = interpolate(single(5),single(0),single(20),single(1),single(t_pnum));
    LM_VSLRearPath3Qulity = single(t_quality * t_factor);
    LM_VSLRearPath1P = LM_VSLRearPath3P;
    LM_VSLRearPath1Qulity = single(0.95);
    LM_VSLRearPath2P = LM_VSLRearPath3P;
    LM_VSLRearPath2Qulity = single(0.95);
    t_dc0 = single(0-LM_VSLRearPath1P(4));
    LM_VSLRearPath1P(4) = single(0);
    LM_VSLRearPath2P(4) = single(LM_VSLRearPath2P(4)+t_dc0);
    LM_VSLRearPath3P(4) = single(LM_VSLRearPath3P(4)+t_dc0);
    else
%%后方第一段拟合  
    t_fity1_end = single(0);
    t_fity2_start = single(0);
    t_fity2_end = single(0);
    t_fity3_start = single(0);
    t_pnum = uint8(0);
for i = 1:t_fornum
    if abs(LM_VSLC0HistInfoX(t_index(i))) <= abs(LM_RearPath1Dis)
        t_pnum = t_pnum + 1;
        if LM_VSLC0BufferDis==255
           t_hpx(t_pnum) = LM_VSLC0HistInfoX(t_index(i));
           t_hpy(t_pnum) = LM_VSLC0HistInfoY(t_index(i));
        end
    end
end
if t_pnum ~=0
      if t_pnum < P_LM_EMLHPFitBuffSize 
        for i = t_pnum+1:P_LM_EMLHPFitBuffSize
            t_hpx(i) = t_hpx(t_pnum);
           t_hpy(i) = t_hpy(t_pnum);
        end
      end

      t = uint8(10);
      z = single(zeros(1,2));
      I = single(zeros(1,2));
      t_x=single(zeros(t,1));
      t_y=single(zeros(t,1));
      for i=1:t
          z(1) = t_hpx(2*i-1);
          z(2) = t_hpx(2*i);
          t_x(i) = mean(z);
          I(1) = t_hpy(2*i-1);
          I(2) = t_hpy(2*i);
          t_y(i)=mean(I);
      end
     x =t_y;
     t_y = hampel(x);
    % 第1段参数拟合
    LM_VSLRearPath1P = polyfit(t_x,t_y,3);
    % 第一段拟合误差计算
    t_fity = polyval(LM_VSLRearPath1P,t_x);
    t_sumerry = single(0);
    for i=1:t
        t_erry = single((t_y(i) - t_fity(i))^2);
        t_sumerry = t_sumerry + t_erry;
    end
    t_quality = interpolate(single(0.5),single(1),single(3),single(0),single(t_sumerry));
    t_factor = interpolate(single(5),single(0),single(17),single(1),single(t_pnum));
    LM_VSLRearPath1Qulity = single(t_quality * t_factor);
     t_fity1_end = polyval(LM_VSLRearPath1P,-30);
    if isnan( LM_VSLRearPath1P(1))
        LM_VSLRearPath1P = single([0 0 0 0]);
        LM_VSLRearPath1Qulity = single(0);
     end   
else 
    LM_VSLRearPath1P = single([0 0 0 0]);
    LM_VSLRearPath1Qulity = single(0);
   
end
LM_EMLHistMaxDis = abs(LM_VSLLRC0HistInfoX(LM_EMLHistPFristPos));
%% 后方第二段轨迹拟合
if LM_EMLHistMaxDis > abs(LM_RearPath1Dis)+10
    t_pnum = uint8(0);
    for i = 1:t_fornum
        if abs(LM_VSLLRC0HistInfoX(t_index(i))) > abs(LM_RearPath1Dis)-6 && abs(LM_VSLLRC0HistInfoX(t_index(i))) <= abs(LM_RearPath2Dis)
            t_pnum = t_pnum + 1;
            if LM_VSLC0BufferDis==255
               t_hpx(t_pnum) = LM_VSLC0HistInfoX(t_index(i));
               t_hpy(t_pnum) = LM_VSLC0HistInfoY(t_index(i));
           end
        end
   end
    if t_pnum < P_LM_EMLHPFitBuffSize
        for i = t_pnum+1:P_LM_EMLHPFitBuffSize
            t_hpx(i) = t_hpx(t_pnum);
            t_hpy(i) = t_hpy(t_pnum);
        end
    end
      t = uint8(10);
       z = single(zeros(1,2));
      I = single(zeros(1,2));
      t_x=single(zeros(t,1));
      t_y=single(zeros(t,1));
      for i=1:t
          z(1) = t_hpx(2*i-1);
          z(2) = t_hpx(2*i);
          t_x(i) = mean(z);
          I(1) = t_hpy(2*i-1);
          I(2) = t_hpy(2*i);
          t_y(i)=mean(I);
      end
     x =t_y;
     t_y = hampel(x);
    % 第2段参数拟合
    LM_VSLRearPath2P = polyfit(t_x,t_y,3);
    % 第2段拟合误差计算
    t_fity = polyval(LM_VSLRearPath2P,t_x);
    t_sumerry = single(0);
    for i=1:t
        t_erry = single((t_y(i) - t_fity(i))^2);
        t_sumerry = t_sumerry + t_erry;
    end
    t_quality = interpolate(0.5,1,3,0,t_sumerry);
    t_factor = interpolate(7,0,17,1,t_pnum);
    LM_VSLRearPath2Qulity = single(t_quality * t_factor);
     t_fity2_start = polyval(LM_VSLRearPath2P,-30);
     t_fity2_end = polyval(LM_VSLRearPath2P,-60);
else
    LM_VSLRearPath2P = single([0 0 0 0]);
    LM_VSLRearPath2Qulity = single(0);
end
%% 后方第3段轨迹拟合
if LM_EMLHistMaxDis > abs(LM_RearPath2Dis) + 10
    t_pnum = uint8(0);
    for i = 1:t_fornum
        if abs(LM_VSLLRC0HistInfoX(t_index(i))) > abs(LM_RearPath2Dis)-6 && abs(LM_VSLLRC0HistInfoX(t_index(i))) <= abs(LM_RearPath3Dis)
            t_pnum = t_pnum + 1;
            if LM_VSLC0BufferDis==255
               t_hpx(t_pnum) = LM_VSLC0HistInfoX(t_index(i));
               t_hpy(t_pnum) = LM_VSLC0HistInfoY(t_index(i));
           end
        end
   end
    if t_pnum < P_LM_EMLHPFitBuffSize
        for i = t_pnum+1:P_LM_EMLHPFitBuffSize
            t_hpx(i) = t_hpx(t_pnum);
            t_hpy(i) = t_hpy(t_pnum);
        end
    end
      t = uint8(10);
       z = single(zeros(1,2));
      I = single(zeros(1,2));
      t_x=single(zeros(t,1));
      t_y=single(zeros(t,1));
      for i=1:t
          z(1) = t_hpx(2*i-1);
          z(2) = t_hpx(2*i);
          t_x(i) = mean(z);
          I(1) = t_hpy(2*i-1);
          I(2) = t_hpy(2*i);
          t_y(i)=mean(I);
      end
     x =t_y;
     t_y = hampel(x);
    % 第3段参数拟合
    LM_VSLRearPath3P = polyfit(t_x,t_y,3);
    % 第3段拟合误差计算
    t_fity = polyval(LM_VSLRearPath3P,t_x);
    t_sumerry = single(0);
    for i=1:t
        t_erry = single((t_y(i) - t_fity(i))^2);
        t_sumerry = t_sumerry + t_erry;
    end
    %由拟合误差求轨迹quality，当拟合误差小于0.5时，轨迹质量为1；当拟合误差大于3时，轨迹质量为0，否则轨迹质量插值
    t_quality = interpolate(single(0.5),single(1),single(3),single(0),single(t_sumerry));
    %由轨迹点个数求轨迹质量影响因子，当轨迹点小于4个时，轨迹质量影响因子为0；当轨迹点大于8个时，轨迹质量影响因子为1
    t_factor = interpolate(single(4),single(0),single(8),single(1),single(t_pnum));
    %轨迹质量= 轨迹质量*轨迹质量影响因子
    LM_VSLRearPath3Qulity = single(t_quality * t_factor);
     LM_VSLRearPath3Qulity = min(LM_VSLRearPath3Qulity,0.95);
      t_fity3_start = polyval(LM_VSLRearPath3P,-60);
     % LM_EMLRearPath3Qulity = single(0); 
else
    LM_VSLRearPath3P = single([0 0 0 0]);
    LM_VSLRearPath3Qulity = single(0);
end

deta1 = t_fity1_end - t_fity2_start;
deta2 = t_fity2_end - t_fity3_start;
if deta1 > 0.2 ||deta1 < -0.2 || deta2 > 0.2 || deta2 < -0.2
t_dc0 = single(0-LM_VSLRearPath1P(4));
LM_VSLRearPath1P(4) = single(0);
LM_VSLRearPath2P(4) = single(LM_VSLRearPath2P(4)+t_dc0+deta1);
LM_VSLRearPath3P(4) = single(LM_VSLRearPath3P(4)+t_dc0+deta1+deta2);
else
LM_VSLRearPath1P(4) = single(0);
LM_VSLRearPath2P(4) = single(LM_VSLRearPath2P(4));
LM_VSLRearPath3P(4) = single(LM_VSLRearPath3P(4));
end
    end
 else 
    LM_VSLRearPath3P = single([0 0 0 0]);
    LM_VSLRearPath3Qulity = single(0);
    LM_VSLRearPath1P = single([0 0 0 0]);
    LM_VSLRearPath1Qulity = single(0);
    LM_VSLRearPath2P = single([0 0 0 0]);
    LM_VSLRearPath2Qulity = single(0);
end
end
%%
function out = interpolate(x1,z1,x2,z2,Raw)
if Raw<=x1
    out = single(z1);
else
    if Raw>=x2
        out = single(z2);
    else
        t_out = single((Raw-x1)*(z2-z1));
        t_out = single(t_out/(x2-x1));
        t_out = single(z1)+t_out;
        out = t_out;
    end
end
end
function out = hampel(x)
% lx = length(x);
lx = uint8(10);
% k = 2;
% iLo = (1:lx)-k;
% iHi = (1:lx)+k;
% iLo(iLo<1) = 1;
% iHi(iHi>lx) = lx;
mmed = zeros(lx,1);
mmad = zeros(lx,1);
w = single(zeros(5,1));
for j = 1:lx
    if j < 3
       medj = x(j);
    elseif j > 8
        medj = x(j);
    else
            w(1) = x(j-2);
            w(2) = x(j-1);
            w(3) = x(j);
            w(4) = x(j+1);
            w(5) = x(j+2);
%             w1 = x(Lo(j):Hi(j));
            medj = median(w);
    end
%     w = x(iLo(j):iHi(j));
%     medj = median(w);
    mmed(j) = medj;
    mmad(j) = median(abs(w-medj));
end
out = mmed;
end
function out = hampel1(x)
% lx = length(x);
lx1 = uint8(20);
% k = 2;
% Lo = (1:lx1)-k;
% Hi = (1:lx1)+k;
% Lo(Lo<1) = 1;
% Hi(Hi>lx1) = lx1;
mmed = zeros(lx1,1);
mmad = zeros(lx1,1);
w1 = single(zeros(5,1));
for j = 1:lx1
    if j < 3
       medj = x(j);
    elseif j > 18
        medj = x(j);
    else
            w1(1) = x(j-2);
            w1(2) = x(j-1);
            w1(3) = x(j);
            w1(4) = x(j+1);
            w1(5) = x(j+2);
%             w1 = x(Lo(j):Hi(j));
            medj = median(w1);
    end
            
            mmed(j) = medj;
            mmad(j) = median(abs(w1-medj));
end
out = mmed;
end

== matlab function PubIfDecisionLM_MDL/Subsystem2/LM_Fusion1/LM_FusBaseLineInfoCalc/LM_FusBLFntPath1130/LM_EVOFFntPath3/LM_FusBLPathC1Calc/MATLAB Function ==
  data: u1 input; y output; yk1 input
function y = fcn(u1,yk1)
y = single(u1);
if isnan(u1)
    if isnan(yk1)
        y = single(0);
    else
        if yk1 ~= 0
            y = single(yk1);
        else
            y = single(0);
        end
    end
end

== matlab function PubIfDecisionLM_MDL/Subsystem2/LM_Fusion1/LM_FusBaseLineInfoCalc/LM_FusBLFntPath1130/LM_EVOFFntPath3/LM_FusBLPathC2Calc/MATLAB Function ==
  data: u1 input; y output; yk1 input
function y = fcn(u1,yk1)
y = single(u1);
if isnan(u1)
    if isnan(yk1)
        y = single(0);
    else
        if yk1 ~= 0
            y = single(yk1);
        else
            y = single(0);
        end
    end
end

== matlab function PubIfDecisionLM_MDL/Subsystem2/LM_Fusion1/LM_FusBaseLineInfoCalc/LM_FusBLFntPath1130/LM_EVOFFntPath3/LM_FusBLPathC3Calc/MATLAB Function ==
  data: u1 input; y output; yk1 input
function y = fcn(u1,yk1)
y = single(u1);
if isnan(u1)
    if isnan(yk1)
        y = single(0);
    else
        if yk1 ~= 0
            y = single(yk1);
        else
            y = single(0);
        end
    end
end

== stateflow chart PubIfDecisionLM_MDL/Subsystem2/LM_Fusion1/LM_FusBaseLineInfoCalc/LM_FusBLFntPath1130/LM_EVOFFntPath3/LM_FusBLPathQualityCalc ==
  state PathDisappear
    en:
    LM_FusBLPathQuality = single(0);
    du:
    LM_FusBLPathQuality = single(0);
    ex:
    LM_FusBLPathQuality = single(0);
  state PathMid2Appear
    en:
    t_times = uint8(0);
    LM_FusBLPathQuality = single(0);
    du:
    t_times = t_times + uint8(1);
    LM_FusBLPathQuality = single(0);
  state PathMid2Disappear
    en:
    t_times = uint8(0);
    LM_FusBLPathQuality = LM_FusPathEMLK * LM_EMLPathQuality + LM_FusPathVSLK * LM_VSLPathQuality + LM_FusPathOTLK * LM_OTLPathQuality;
    du:
    t_times = t_times + uint8(1);
    LM_FusBLPathQuality = LM_FusPathEMLK * LM_EMLPathQuality + LM_FusPathVSLK * LM_VSLPathQuality + LM_FusPathOTLK * LM_OTLPathQuality;
  state PathAppear
    en:
    LM_FusBLPathQuality = LM_FusPathEMLK * LM_EMLPathQuality + LM_FusPathVSLK * LM_VSLPathQuality + LM_FusPathOTLK * LM_OTLPathQuality;
    du:
    LM_FusBLPathQuality = LM_FusPathEMLK * LM_EMLPathQuality + LM_FusPathVSLK * LM_VSLPathQuality + LM_FusPathOTLK * LM_OTLPathQuality;
  (default) -> PathDisappear
  PathMid2Disappear -> PathDisappear [order 2] : [(LM_EMLPathQuality == 0 && LM_VSLPathQuality == 0 && LM_OTLPathQuality == 0) && t_times > 10]
  PathDisappear -> PathMid2Appear : [LM_EMLPathQuality ~= 0 || LM_VSLPathQuality ~= 0 || LM_OTLPathQuality ~= 0]
  PathMid2Appear -> PathDisappear [order 1] : [LM_EMLPathQuality == 0 && LM_VSLPathQuality == 0 && LM_OTLPathQuality == 0]
  PathMid2Appear -> PathAppear [order 2] : [(LM_EMLPathQuality ~= 0 || LM_VSLPathQuality ~= 0 || LM_OTLPathQuality ~= 0) && t_times > uint8(5)]
  PathMid2Disappear -> PathAppear [order 1] : [LM_EMLPathQuality ~= 0 || LM_VSLPathQuality ~= 0 || LM_OTLPathQuality ~= 0]
  PathAppear -> PathMid2Disappear : [LM_EMLPathQuality == 0 && LM_VSLPathQuality == 0 && LM_OTLPathQuality == 0]
  data: LM_EMLPathQuality input; LM_VSLPathQuality input; LM_OTLPathQuality input; LM_FusPathEMLK input; LM_FusPathVSLK input; LM_FusPathOTLK input; LM_FusBLPathQuality output single size=1; t_times local uint8 size=1

== matlab function PubIfDecisionLM_MDL/Subsystem2/LM_Fusion1/LM_FusBaseLineInfoCalc/LM_FusBLFntPath1130/LM_EVOFFntPath2/LM_FusBLPathC1Calc/MATLAB Function ==
  data: u1 input; y output; yk1 input
function y = fcn(u1,yk1)
y = single(u1);
if isnan(u1)
    if isnan(yk1)
        y = single(0);
    else
        if yk1 ~= 0
            y = single(yk1);
        else
            y = single(0);
        end
    end
end

== matlab function PubIfDecisionLM_MDL/Subsystem2/LM_Fusion1/LM_FusBaseLineInfoCalc/LM_FusBLFntPath1130/LM_EVOFFntPath2/LM_FusBLPathC2Calc/MATLAB Function ==
  data: u1 input; y output; yk1 input
function y = fcn(u1,yk1)
y = single(u1);
if isnan(u1)
    if isnan(yk1)
        y = single(0);
    else
        if yk1 ~= 0
            y = single(yk1);
        else
            y = single(0);
        end
    end
end

== matlab function PubIfDecisionLM_MDL/Subsystem2/LM_Fusion1/LM_FusBaseLineInfoCalc/LM_FusBLFntPath1130/LM_EVOFFntPath2/LM_FusBLPathC3Calc/MATLAB Function ==
  data: u1 input; y output; yk1 input
function y = fcn(u1,yk1)
y = single(u1);
if isnan(u1)
    if isnan(yk1)
        y = single(0);
    else
        if yk1 ~= 0
            y = single(yk1);
        else
            y = single(0);
        end
    end
end

== stateflow chart PubIfDecisionLM_MDL/Subsystem2/LM_Fusion1/LM_FusBaseLineInfoCalc/LM_FusBLFntPath1130/LM_EVOFFntPath2/LM_FusBLPathQualityCalc ==
  state PathDisappear
    en:
    LM_FusBLPathQuality = single(0);
    du:
    LM_FusBLPathQuality = single(0);
    ex:
    LM_FusBLPathQuality = single(0);
  state PathMid2Appear
    en:
    t_times = uint8(0);
    LM_FusBLPathQuality = single(0);
    du:
    t_times = t_times + uint8(1);
    LM_FusBLPathQuality = single(0);
  state PathMid2Disappear
    en:
    t_times = uint8(0);
    LM_FusBLPathQuality = LM_FusPathEMLK * LM_EMLPathQuality + LM_FusPathVSLK * LM_VSLPathQuality + LM_FusPathOTLK * LM_OTLPathQuality;
    du:
    t_times = t_times + uint8(1);
    LM_FusBLPathQuality = LM_FusPathEMLK * LM_EMLPathQuality + LM_FusPathVSLK * LM_VSLPathQuality + LM_FusPathOTLK * LM_OTLPathQuality;
  state PathAppear
    en:
    LM_FusBLPathQuality = LM_FusPathEMLK * LM_EMLPathQuality + LM_FusPathVSLK * LM_VSLPathQuality + LM_FusPathOTLK * LM_OTLPathQuality;
    du:
    LM_FusBLPathQuality = LM_FusPathEMLK * LM_EMLPathQuality + LM_FusPathVSLK * LM_VSLPathQuality + LM_FusPathOTLK * LM_OTLPathQuality;
  (default) -> PathDisappear
  PathMid2Disappear -> PathDisappear [order 2] : [(LM_EMLPathQuality == 0 && LM_VSLPathQuality == 0 && LM_OTLPathQuality == 0) && t_times > 10]
  PathDisappear -> PathMid2Appear : [LM_EMLPathQuality ~= 0 || LM_VSLPathQuality ~= 0 || LM_OTLPathQuality ~= 0]
  PathMid2Appear -> PathDisappear [order 1] : [LM_EMLPathQuality == 0 && LM_VSLPathQuality == 0 && LM_OTLPathQuality == 0]
  PathMid2Appear -> PathAppear [order 2] : [(LM_EMLPathQuality ~= 0 || LM_VSLPathQuality ~= 0 || LM_OTLPathQuality ~= 0) && t_times > uint8(5)]
  PathMid2Disappear -> PathAppear [order 1] : [LM_EMLPathQuality ~= 0 || LM_VSLPathQuality ~= 0 || LM_OTLPathQuality ~= 0]
  PathAppear -> PathMid2Disappear : [LM_EMLPathQuality == 0 && LM_VSLPathQuality == 0 && LM_OTLPathQuality == 0]
  data: LM_EMLPathQuality input; LM_VSLPathQuality input; LM_OTLPathQuality input; LM_FusPathEMLK input; LM_FusPathVSLK input; LM_FusPathOTLK input; LM_FusBLPathQuality output single size=1; t_times local uint8 size=1
